simulink model "identificacion"  (R2018a)
settings: Solver=VariableStepAuto  StartTime=0.0  StopTime=1000  RelTol=1e-3
undefined symbols (not defined in the file or in its folder): tf3
settings Model: Creator=carma  LastModifiedBy=carma

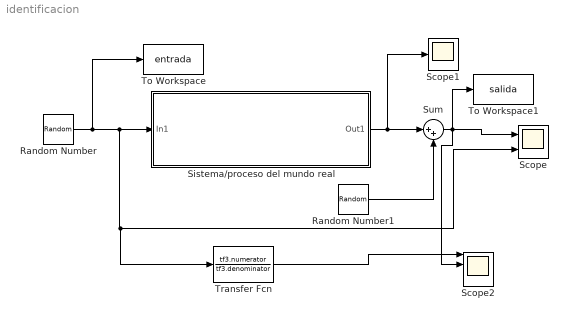
== system identificacion ==
  Random Number : RandomNumber  Variance=0.2  SampleTime=50
  Random Number1 : RandomNumber  Variance=0.015  SampleTime=0.1
  Scope : Scope  NumInputPorts=2
  Scope1 : Scope
  Scope2 : Scope  NumInputPorts=4
  Sistema/proceso del mundo real : Subsystem
  Sum : Sum  Inputs=|++
  To Workspace : ToWorkspace  VariableName=entrada  SampleTime=1
  To Workspace1 : ToWorkspace  VariableName=salida  SampleTime=1
  Transfer Fcn : TransferFcn  Numerator=tf3.numerator  Denominator=tf3.denominator
  wires:
  Random Number1/1 -> Sum/2
  Sistema/proceso del mundo real/1(Out1) -> Scope1/1, Sum/1
  Sum/1 -> Scope2/2, To Workspace1/1, Scope/1
  Random Number/1 -> To Workspace/1, Transfer Fcn/1, Scope/2, Sistema/proceso del mundo real/1(In1)
  Transfer Fcn/1 -> Scope2/1

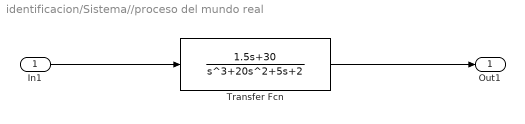
== system identificacion/Sistema//proceso del mundo real ==
  In1 : Inport
  Transfer Fcn : TransferFcn  Numerator=[1.5 30]  Denominator=[1 20 5 2]
  Out1 : Outport
  wires:
  Transfer Fcn/1 -> Out1/1
  In1/1 -> Transfer Fcn/1
